simulink model "poleplacement_controller_and_observer"  (R2016b)
settings: Solver=VariableStepAuto  StartTime=0.0  StopTime=T  RelTol=1e-3
undefined symbols (not defined in the file or in its folder): blackboxie, h, K, L, Nbar
settings Model: Creator=Miranda  LastModifiedBy=Miranda

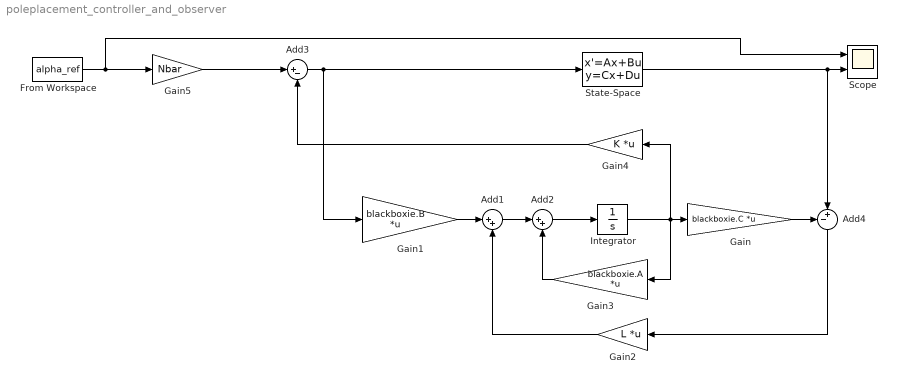
== system poleplacement_controller_and_observer ==
  Add1 : Sum  Inputs=|++
  Add2 : Sum  Inputs=|++
  Add3 : Sum  Inputs=|+-
  Add4 : Sum  Inputs=-+|
  From Workspace : FromWorkspace  VariableName=alpha_ref  SampleTime=h
  Gain : Gain  Gain=blackboxie.C  Multiplication=Matrix(K*u)
  Gain1 : Gain  Gain=blackboxie.B  Multiplication=Matrix(K*u)
  Gain2 : Gain  Gain=L  Multiplication=Matrix(K*u)
  Gain3 : Gain  Gain=blackboxie.A  Multiplication=Matrix(K*u)
  Gain4 : Gain  Gain=K  Multiplication=Matrix(K*u)
  Gain5 : Gain  Gain=Nbar
  Integrator : Integrator
  Scope : Scope  NumInputPorts=2
  State-Space : StateSpace  A=blackboxie.A  B=blackboxie.B  C=blackboxie.C  D=blackboxie.D  X0=0
  wires:
  Gain1/1 -> Add1/1
  Add1/1 -> Add2/1
  Add2/1 -> Integrator/1
  Integrator/1 -> Gain4/1, Gain/1, Gain3/1
  Gain2/1 -> Add1/2
  Gain3/1 -> Add2/2
  Gain/1 -> Add4/1
  Add4/1 -> Gain2/1
  State-Space/1 -> Scope/2, Add4/2
  Add3/1 -> Gain1/1, State-Space/1
  Gain4/1 -> Add3/2
  From Workspace/1 -> Scope/1, Gain5/1
  Gain5/1 -> Add3/1
